simulink model "Noa_Nofusion_backup"  (R2020b)
settings: Solver=FixedStepDiscrete  StartTime=0.0  StopTime=Inf  FixedStep=0.02  RelTol=1e-3
PostLoadFcn:
  | if any(exist('dsrtsu_mdlpostloadfcn', 'file') ~= 0), dsrtsu_mdlpostloadfcn('Execute', bdroot); end
InitFcn:
  | , if any(exist('rtifpga_mdlclblib', 'file') ~= 0), rtifpga_mdlclblib('Init', bdroot); end,
  | , if any(exist('dsmpb_private', 'file') ~= 0), dsmpb_private('dsmpb_mdlclblib', 'Init', bdroot); end,
undefined symbols (not defined in the file): ACC_TimeGap_DecSetSwt, ACC_TimeGap_IncSetSwt, AccelPedalPosn, AccelPedalPosnVldty, AccelPedlPosnDiagc, AccPedalOverride, ACU_ShiftInProgress, ADAS_Posn_CurLane, AESSwtReq, ALC_SwtReq, BrkPedalSts, CC_ACC_CANCEL_OFFSwt, CC_ACC_CRUISE_OFFSwt, CC_ACC_DecSetSpd_SetSwt, CC_ACC_IncSetSpd_ResuSwt, CC_ACCSwtErr, CharSpd_ms, CSA_NODE, CURRENT_GEAR, CurrentGearValid, DiscIntNeverNeededParam, DrvDoorSts, DrvSBR, DrvTrqReqOvld, ECMACCInterface, ECMRespACC, ELKSwtReq, EngLimpHomeSts, EngSpd, EngState, EngState_PHEV, EngTrqMaxActSpd, EngTrqMinAct, EPS_DrvInpTrqVal_HighReslolution, EPS_FailSts, EPS_LKATorqOvrlDlvd, EPS_LKATorqOvrlDlvdVld, EPS_LKATrqOvlDlvdSts, EPS_SteerMod, EPS_TrqSnsrSts, EQ4_APPINFO, EQ4_LA_ELEM, EQ4_LA_HDR, EQ4_LAP_ELEM, EQ4_LAP_HDR, EQ4_LH_ELEM, EQ4_LH_HDR, EQ4_LRE_ELEM, EQ4_LRE_HDR, ESS_PedSwtReq, ESS_VehSwtReq, FFogLmpSts_F_Pbox, FLWheelDriveDirection, FLWheelSpd, FrntWiprSwtSts, FrntWshrSwtSts, FRWheelDriveDirection, FRWheelSpd, HazardLmpSwtSts, HCU_AccelPedalPosn_Diag ... (+152)
libraries: simulink x117, dsmpblib x30
(part 7 of 11)

== system Noa_Nofusion_backup/Common/Subsystem7/DS ==
  canDMSSts : Inport  OutDataTypeStr=uint8
  canHeadDetn : Inport  Port=2  OutDataTypeStr=boolean
  canDistrctnLevel : Inport  Port=3  OutDataTypeStr=uint8
  canDistrctnQlty : Inport  Port=4  OutDataTypeStr=uint8
  canDrowsnsLevel : Inport  Port=5  OutDataTypeStr=uint8
  DriverStsConditnJudge : Subsystem
  DriverSts_StateMachine : Stateflow chart  TreatAsAtomicUnit=on
  P_DMS_tDSGoodUnbeliv2LowDistrctn : Constant  Value=P_DMS_tDSGoodUnbeliv2LowDistrctn
  P_DMS_tDSGoodUnbeliv2LowDrowsns : Constant  Value=P_DMS_tDSGoodUnbeliv2LowDrowsns
  P_DMS_tDSGoodUnbeliv2MidDistractn : Constant  Value=P_DMS_tDSGoodUnbeliv2MidDistractn
  P_DMS_tDSGoodUnbeliv2MidDrowsns : Constant  Value=P_DMS_tDSGoodUnbeliv2MidDrowsns
  P_DMS_tDSLow2MidDistractn : Constant  Value=P_DMS_tDSLow2MidDistractn
  P_DMS_tDSLow2MidDrowsns : Constant  Value=P_DMS_tDSLow2MidDrowsns
  P_DMS_tDSOther2Hi1Distractn : Constant  Value=P_DMS_tDSOther2Hi1Distractn
  P_DMS_tDSOther2Hi1Drowsns : Constant  Value=P_DMS_tDSOther2Hi1Drowsns
  P_DMS_tDSOther2Hi2Distractn : Constant  Value=P_DMS_tDSOther2Hi2Distractn
  P_DMS_tDSOther2Hi2Drowsns : Constant  Value=P_DMS_tDSOther2Hi2Drowsns
  DistractnSts : Outport  OutDataTypeStr=uint8
  DrowsnsSts : Outport  Port=2  OutDataTypeStr=uint8
  DriverSts : Outport  Port=3  OutDataTypeStr=uint8
  wires:
  canDistrctnLevel/1 -> DriverStsConditnJudge/3(canDistrctnLevel)
  canDistrctnQlty/1 -> DriverStsConditnJudge/4(canDistrctnQlty)
  canHeadDetn/1 -> DriverStsConditnJudge/2(canHeadDetn)
  canDrowsnsLevel/1 -> DriverStsConditnJudge/5(canDrowsnsLevel)
  canDMSSts/1 -> DriverStsConditnJudge/1(canDMSSts)
  P_DMS_tDSGoodUnbeliv2LowDistrctn/1 -> DriverStsConditnJudge/6(PtDSGoodUnbeliv2LowDistrctn)
  P_DMS_tDSGoodUnbeliv2MidDistractn/1 -> DriverStsConditnJudge/7(PtDSGoodUnbeliv2MidDistractn)
  P_DMS_tDSLow2MidDistractn/1 -> DriverStsConditnJudge/8(PtDSLow2MidDistractn)
  P_DMS_tDSOther2Hi1Distractn/1 -> DriverStsConditnJudge/9(PtDSOther2Hi1Distractn)
  P_DMS_tDSOther2Hi2Distractn/1 -> DriverStsConditnJudge/10(PtDSOther2Hi2Distractn)
  P_DMS_tDSGoodUnbeliv2LowDrowsns/1 -> DriverStsConditnJudge/11(PtDSGoodUnbeliv2LowDrowsns)
  P_DMS_tDSGoodUnbeliv2MidDrowsns/1 -> DriverStsConditnJudge/12(PtDSGoodUnbeliv2MidDrowsns)
  P_DMS_tDSLow2MidDrowsns/1 -> DriverStsConditnJudge/13(PtDSLow2MidDrowsns)
  P_DMS_tDSOther2Hi1Drowsns/1 -> DriverStsConditnJudge/14(PtDSOther2Hi1Drowsns)
  P_DMS_tDSOther2Hi2Drowsns/1 -> DriverStsConditnJudge/15(PtDSOther2Hi2Drowsns)
  DriverStsConditnJudge/1(DSOther2Good) -> DriverSts_StateMachine/1(DSOther2Good)
  DriverStsConditnJudge/2(DSOther2Unbeliv) -> DriverSts_StateMachine/2(DSOther2Unbeliv)
  DriverStsConditnJudge/3(DSGoodUnbeliv2LowDistractn) -> DriverSts_StateMachine/3(DSGoodUnbeliv2LowDistractn)
  DriverStsConditnJudge/4(DSMidHi1Hi22LowDistractn) -> DriverSts_StateMachine/4(DSMidHi1Hi22LowDistractn)
  DriverStsConditnJudge/5(DSGoodUnbeliv2MidDistractn) -> DriverSts_StateMachine/5(DSGoodUnbeliv2MidDistractn)
  DriverStsConditnJudge/6(DSLow2MidDistractn) -> DriverSts_StateMachine/6(DSLow2MidDistractn)
  DriverStsConditnJudge/7(DSHi1Hi22MidDistractn) -> DriverSts_StateMachine/7(DSHi1Hi22MidDistractn)
  DriverStsConditnJudge/8(DSOther2Hi1Distractn) -> DriverSts_StateMachine/8(DSOther2Hi1Distractn)
  DriverStsConditnJudge/9(DSOther2Hi2Distractn) -> DriverSts_StateMachine/9(DSOther2Hi2Distractn)
  DriverStsConditnJudge/10(DSGoodUnbeliv2LowDrowsns) -> DriverSts_StateMachine/10(DSGoodUnbeliv2LowDrowsns)
  DriverStsConditnJudge/11(DSMidHi1Hi22LowDrowsns) -> DriverSts_StateMachine/11(DSMidHi1Hi22LowDrowsns)
  DriverStsConditnJudge/12(DSGoodUnbeliv2MidDrowsns) -> DriverSts_StateMachine/12(DSGoodUnbeliv2MidDrowsns)
  DriverStsConditnJudge/13(DSLow2MidDrowsns) -> DriverSts_StateMachine/13(DSLow2MidDrowsns)
  DriverStsConditnJudge/14(DSHi1Hi22MidDrowsns) -> DriverSts_StateMachine/14(DSHi1Hi22MidDrowsns)
  DriverStsConditnJudge/15(DSOther2Hi1Drowsns) -> DriverSts_StateMachine/15(DSOther2Hi1Drowsns)
  DriverStsConditnJudge/16(DSOther2Hi2Drowsns) -> DriverSts_StateMachine/16(DSOther2Hi2Drowsns)
  DriverStsConditnJudge/17(DSMidHi1Hi22NoDistractn) -> DriverSts_StateMachine/17(DSMidHi1Hi22NoDistractn)
  DriverStsConditnJudge/18(DSMidHi1Hi22NoDrowsns) -> DriverSts_StateMachine/18(DSMidHi1Hi22NoDrowsns)
  DriverStsConditnJudge/19(DSUnbeliv2DDAEnable) -> DriverSts_StateMachine/19(DSUnbeliv2DDAEnable)
  DriverSts_StateMachine/1(DistractnSts) -> DistractnSts/1
  DriverSts_StateMachine/2(DrowsnsSts) -> DrowsnsSts/1
  DriverSts_StateMachine/3(DriverSts) -> DriverSts/1

== system Noa_Nofusion_backup/LPV/Subsystem5/For Each Subsystem1 ==
  In1 : Inport  Partition=on  PartitionDimension=1  PartitionWidth=1  PartitionOffset=0
  Bus Assignment4 : BusAssignment  AssignedSignals=LH_CRC,LH_Is_Triggered_SDM_Type,LH_Is_Triggered_SDM_Model,LH_Track_ID,LH_Age,LH_Confidence,Reserved_3,LH_Prediction_Reason,LH_Availability_State,LH_Color,LH_Color_Confidence,LH_Lanemark_Type,LH_DLM_Type,LH_DECEL_Type,Reserved_4,LH_Lanemark_Type_Conf,LH_Side,LH_Crossing,LH_Marker_Width,LH_Marker_Width_STD,Reserved_5,LH_Dash_Average_Length,LH_Dash_Average_Gap,LH_Is_Multi_Clothoid,Reserved_6,LH_Line_First_C0,LH_Line_First_C1,LH_Line_First_C2,LH_Line_First_C3,LH_First_VR_Start,LH_First_VR_End,Reserved_7,LH_First_Measured_VR_End,LH_Second_Measured_VR_End,Reserved_8,LH_Line_Second_C0,LH_Line_Second_C1,LH_Line_Second_C2,LH_Line_Second_C3,LH_Second_VR_Start,LH_Second_VR_End,LH_Buffer_C3
  Bus Selector : BusSelector  OutputSignals=LH_CRC,LH_Is_Triggered_SDM_Type,LH_Is_Triggered_SDM_Model,LH_Track_ID,LH_Age,LH_Confidence,Reserved_3,LH_Prediction_Reason,LH_Availability_State,LH_Color,LH_Color_Confidence,LH_Lanemark_Type,LH_DLM_Type,LH_DECEL_Type,Reserved_4,LH_Lanemark_Type_Conf,LH_Side,LH_Crossing,LH_Marker_Width,LH_Marker_Width_STD,Reserved_5,LH_Dash_Average_Length,LH_Dash_Average_Gap,LH_Is_Multi_Clothoid,Reserved_6,LH_Line_First_C0,LH_Line_First_C1,LH_Line_First_C2,LH_Line_First_C3,LH_First_VR_Start,LH_First_VR_End,Reserved_7,LH_First_Measured_VR_End,LH_Second_Measured_VR_End,Reserved_8,LH_Line_Second_C0,LH_Line_Second_C1,LH_Line_Second_C2,LH_Line_Second_C3,LH_Second_VR_Start,LH_Second_VR_End,LH_Buffer_C3
  Constant4 : Constant  Value=0  OutDataTypeStr=Bus: EQ4_LH_ELEM_BUS
  For Each : ForEach  DisableCoverage=on
  Out1 : Outport  ConcatenationDimension=1
  wires:
  Bus Selector/42 -> Bus Assignment4/43  "<LH_Buffer_C3>"
  Bus Selector/41 -> Bus Assignment4/42  "<LH_Second_VR_End>"
  Bus Selector/40 -> Bus Assignment4/41  "<LH_Second_VR_Start>"
  Bus Selector/39 -> Bus Assignment4/40  "<LH_Line_Second_C3>"
  Bus Selector/38 -> Bus Assignment4/39  "<LH_Line_Second_C2>"
  Bus Selector/37 -> Bus Assignment4/38  "<LH_Line_Second_C1>"
  Bus Selector/36 -> Bus Assignment4/37  "<LH_Line_Second_C0>"
  Bus Selector/35 -> Bus Assignment4/36  "<Reserved_8>"
  Bus Selector/34 -> Bus Assignment4/35  "<LH_Second_Measured_VR_End>"
  Bus Selector/33 -> Bus Assignment4/34  "<LH_First_Measured_VR_End>"
  Bus Selector/32 -> Bus Assignment4/33  "<Reserved_7>"
  Bus Selector/31 -> Bus Assignment4/32  "<LH_First_VR_End>"
  Bus Selector/30 -> Bus Assignment4/31  "<LH_First_VR_Start>"
  Bus Selector/29 -> Bus Assignment4/30  "<LH_Line_First_C3>"
  Bus Selector/28 -> Bus Assignment4/29  "<LH_Line_First_C2>"
  Bus Selector/27 -> Bus Assignment4/28  "<LH_Line_First_C1>"
  Bus Selector/26 -> Bus Assignment4/27  "<LH_Line_First_C0>"
  Bus Selector/25 -> Bus Assignment4/26  "<Reserved_6>"
  Bus Selector/24 -> Bus Assignment4/25  "<LH_Is_Multi_Clothoid>"
  Bus Selector/23 -> Bus Assignment4/24  "<LH_Dash_Average_Gap>"
  Bus Selector/22 -> Bus Assignment4/23  "<LH_Dash_Average_Length>"
  Bus Selector/21 -> Bus Assignment4/22  "<Reserved_5>"
  Bus Selector/20 -> Bus Assignment4/21  "<LH_Marker_Width_STD>"
  Bus Selector/19 -> Bus Assignment4/20  "<LH_Marker_Width>"
  Bus Selector/18 -> Bus Assignment4/19  "<LH_Crossing>"
  Bus Selector/17 -> Bus Assignment4/18  "<LH_Side>"
  Bus Selector/16 -> Bus Assignment4/17  "<LH_Lanemark_Type_Conf>"
  Bus Selector/15 -> Bus Assignment4/16  "<Reserved_4>"
  Bus Selector/14 -> Bus Assignment4/15  "<LH_DECEL_Type>"
  Bus Selector/13 -> Bus Assignment4/14  "<LH_DLM_Type>"
  Bus Selector/12 -> Bus Assignment4/13  "<LH_Lanemark_Type>"
  Bus Selector/11 -> Bus Assignment4/12  "<LH_Color_Confidence>"
  Bus Selector/10 -> Bus Assignment4/11  "<LH_Color>"
  Bus Selector/9 -> Bus Assignment4/10  "<LH_Availability_State>"
  Bus Selector/8 -> Bus Assignment4/9  "<LH_Prediction_Reason>"
  Bus Selector/7 -> Bus Assignment4/8  "<Reserved_3>"
  Bus Selector/6 -> Bus Assignment4/7  "<LH_Confidence>"
  Bus Selector/5 -> Bus Assignment4/6  "<LH_Age>"
  Bus Selector/4 -> Bus Assignment4/5  "<LH_Track_ID>"
  Bus Selector/3 -> Bus Assignment4/4  "<LH_Is_Triggered_SDM_Model>"
  Bus Selector/2 -> Bus Assignment4/3  "<LH_Is_Triggered_SDM_Type>"
  Bus Selector/1 -> Bus Assignment4/2  "<LH_CRC>"
  Bus Assignment4/1 -> Out1/1
  In1/1 -> Bus Selector/1
  Constant4/1 -> Bus Assignment4/1

== system Noa_Nofusion_backup/LPV/Subsystem5/For Each Subsystem2 ==
  In1 : Inport  Partition=on  PartitionDimension=1  PartitionWidth=1  PartitionOffset=0
  Bus Assignment4 : BusAssignment  AssignedSignals=LRE_ID,LRE_Age,LRE_Confidence,LRE_Type,Reserved_2,LRE_Prediction_Reason,LRE_Availability_State,LRE_Height,LRE_Height_STD,Reserved_3,LRE_View_Range_Start,LRE_View_Range_End,Reserved_4,LRE_Measured_VR_End,LRE_Side,LRE_Is_Triggered_SDM_Model,Reserved_5,LRE_Line_C3,LRE_Line_C2,LRE_Line_C1,LRE_Line_C0,LRE_Detection_Source,Reserved_6
  Bus Selector : BusSelector  OutputSignals=LRE_ID,LRE_Age,LRE_Confidence,LRE_Type,Reserved_2,LRE_Prediction_Reason,LRE_Availability_State,LRE_Height,LRE_Height_STD,Reserved_3,LRE_View_Range_Start,LRE_View_Range_End,Reserved_4,LRE_Measured_VR_End,LRE_Side,LRE_Is_Triggered_SDM_Model,Reserved_5,LRE_Line_C3,LRE_Line_C2,LRE_Line_C1,LRE_Line_C0,LRE_Detection_Source,Reserved_6
  Constant4 : Constant  Value=0  OutDataTypeStr=Bus: EQ4_LRE_ELEM_BUS
  For Each : ForEach  DisableCoverage=on
  Out1 : Outport  ConcatenationDimension=1
  wires:
  Bus Selector/23 -> Bus Assignment4/24  "<Reserved_6>"
  Bus Selector/22 -> Bus Assignment4/23  "<LRE_Detection_Source>"
  Bus Selector/21 -> Bus Assignment4/22  "<LRE_Line_C0>"
  Bus Selector/20 -> Bus Assignment4/21  "<LRE_Line_C1>"
  Bus Selector/19 -> Bus Assignment4/20  "<LRE_Line_C2>"
  Bus Selector/18 -> Bus Assignment4/19  "<LRE_Line_C3>"
  Bus Selector/17 -> Bus Assignment4/18  "<Reserved_5>"
  Bus Selector/16 -> Bus Assignment4/17  "<LRE_Is_Triggered_SDM_Model>"
  Bus Selector/15 -> Bus Assignment4/16  "<LRE_Side>"
  Bus Selector/14 -> Bus Assignment4/15  "<LRE_Measured_VR_End>"
  Bus Selector/13 -> Bus Assignment4/14  "<Reserved_4>"
  Bus Selector/12 -> Bus Assignment4/13  "<LRE_View_Range_End>"
  Bus Selector/11 -> Bus Assignment4/12  "<LRE_View_Range_Start>"
  Bus Selector/10 -> Bus Assignment4/11  "<Reserved_3>"
  Bus Selector/9 -> Bus Assignment4/10  "<LRE_Height_STD>"
  Bus Selector/8 -> Bus Assignment4/9  "<LRE_Height>"
  Bus Selector/7 -> Bus Assignment4/8  "<LRE_Availability_State>"
  Bus Selector/6 -> Bus Assignment4/7  "<LRE_Prediction_Reason>"
  Bus Selector/5 -> Bus Assignment4/6  "<Reserved_2>"
  Bus Selector/4 -> Bus Assignment4/5  "<LRE_Type>"
  Bus Selector/3 -> Bus Assignment4/4  "<LRE_Confidence>"
  Bus Selector/2 -> Bus Assignment4/3  "<LRE_Age>"
  Bus Selector/1 -> Bus Assignment4/2  "<LRE_ID>"
  Constant4/1 -> Bus Assignment4/1
  In1/1 -> Bus Selector/1
  Bus Assignment4/1 -> Out1/1

== system Noa_Nofusion_backup/LPV/Subsystem5/For Each Subsystem3 ==
  In1 : Inport  Partition=on  PartitionDimension=1  PartitionWidth=1  PartitionOffset=0
  Bus Assignment4 : BusAssignment  AssignedSignals=LA_Lane_Track_ID,LA_Age,LA_Confidence,LA_Color,LA_Color_Conf,LA_Prediction_Reason,LA_Availability_State,LA_View_Range_Start,Reserved_2,LA_View_Range_End,LA_Measured_VR_End,Reserved_3,LA_Lanemark_Type,LA_DLM_Type,LA_Lanemark_Type_Conf,LA_Line_Side,LA_Marker_Width,Reserved_4,LA_Marker_Width_STD,Reserved_5,LA_Line_C3,LA_Line_C2,LA_Line_C1,LA_Line_C0,LH_Buffer_C1,Reserved_6
  Bus Selector : BusSelector  OutputSignals=LA_Lane_Track_ID,LA_Age,LA_Confidence,LA_Color,LA_Color_Conf,LA_Prediction_Reason,LA_Availability_State,LA_View_Range_Start,Reserved_2,LA_View_Range_End,LA_Measured_VR_End,Reserved_3,LA_Lanemark_Type,LA_DLM_Type,LA_Lanemark_Type_Conf,LA_Line_Side,LA_Marker_Width,Reserved_4,LA_Marker_Width_STD,Reserved_5,LA_Line_C3,LA_Line_C2,LA_Line_C1,LA_Line_C0,LH_Buffer_C1,Reserved_6
  Constant4 : Constant  Value=0  OutDataTypeStr=Bus: EQ4_LA_ELEM_BUS
  For Each : ForEach  DisableCoverage=on
  Out1 : Outport  ConcatenationDimension=1
  wires:
  Bus Selector/26 -> Bus Assignment4/27  "<Reserved_6>"
  Bus Selector/25 -> Bus Assignment4/26  "<LH_Buffer_C1>"
  Bus Selector/24 -> Bus Assignment4/25  "<LA_Line_C0>"
  Bus Selector/23 -> Bus Assignment4/24  "<LA_Line_C1>"
  Bus Selector/22 -> Bus Assignment4/23  "<LA_Line_C2>"
  Bus Selector/21 -> Bus Assignment4/22  "<LA_Line_C3>"
  Bus Selector/20 -> Bus Assignment4/21  "<Reserved_5>"
  Bus Selector/19 -> Bus Assignment4/20  "<LA_Marker_Width_STD>"
  Bus Selector/18 -> Bus Assignment4/19  "<Reserved_4>"
  Bus Selector/17 -> Bus Assignment4/18  "<LA_Marker_Width>"
  Bus Selector/16 -> Bus Assignment4/17  "<LA_Line_Side>"
  Bus Selector/15 -> Bus Assignment4/16  "<LA_Lanemark_Type_Conf>"
  Bus Selector/14 -> Bus Assignment4/15  "<LA_DLM_Type>"
  Bus Selector/13 -> Bus Assignment4/14  "<LA_Lanemark_Type>"
  Bus Selector/12 -> Bus Assignment4/13  "<Reserved_3>"
  Bus Selector/11 -> Bus Assignment4/12  "<LA_Measured_VR_End>"
  Bus Selector/10 -> Bus Assignment4/11  "<LA_View_Range_End>"
  Bus Selector/9 -> Bus Assignment4/10  "<Reserved_2>"
  Bus Selector/8 -> Bus Assignment4/9  "<LA_View_Range_Start>"
  Bus Selector/7 -> Bus Assignment4/8  "<LA_Availability_State>"
  Bus Selector/6 -> Bus Assignment4/7  "<LA_Prediction_Reason>"
  Bus Selector/5 -> Bus Assignment4/6  "<LA_Color_Conf>"
  Bus Selector/4 -> Bus Assignment4/5  "<LA_Color>"
  Bus Selector/3 -> Bus Assignment4/4  "<LA_Confidence>"
  Bus Selector/2 -> Bus Assignment4/3  "<LA_Age>"
  Bus Selector/1 -> Bus Assignment4/2  "<LA_Lane_Track_ID>"
  Constant4/1 -> Bus Assignment4/1
  In1/1 -> Bus Selector/1
  Bus Assignment4/1 -> Out1/1

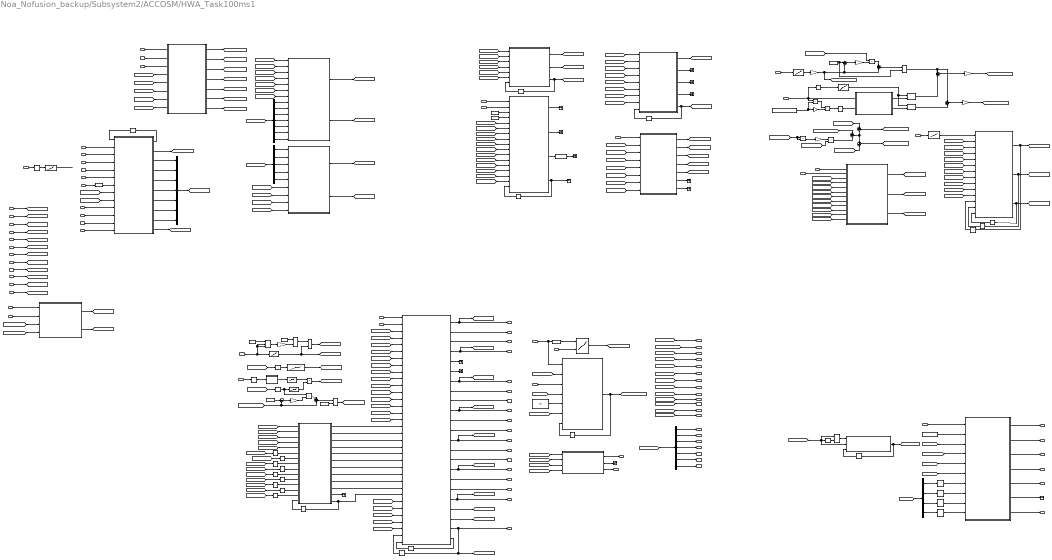
== system Noa_Nofusion_backup/Subsystem2/ACCOSM/HWA_Task100ms1 ==
  note: part03/TOS/Subsystem1/ACCOSM/HWA_Task100ms1
  note: OTL
  note: ATS
  note: PLA
  note: ASI_CalcPreOSF
  note: EIA
  note: 存在时间
  ObjRange_m : Inport
  ObjDx_m : Inport  Port=2
  ObjDy_m : Inport  Port=3
  ObjValid : Inport  Port=4
  ObjClassification : Inport  Port=5
  ObjVxG_ms : Inport  Port=6
  ObjVyG_ms : Inport  Port=7
  ObjArG_ms2 : Inport  Port=8
  ObjWidth_m : Inport  Port=9
  ObjCnt : Inport  Port=10
  ObjMoveSts : Inport  Port=11
  ObjBrakeLightIndic : Inport  Port=12
  A2 : Inport  Port=13
  A1 : Inport  Port=14
  Conf : Inport  Port=15
  TimeGap : Inport  Port=16
  ACCMode : Inport  Port=17
  VxvRef_ms : Inport  Port=18
  kapCurvTraj : Inport  Port=19
  AlpSideSlipAngle : Inport  Port=20
  AlpWheelAngle : Inport  Port=21
  alpSumSlideCurveness : Inport  Port=22
  LongitudeAcc : Inport  Port=23
  TarLineValid : Inport  Port=24
  TarLine_A2 : Inport  Port=25
  TarLine_A1 : Inport  Port=26
  TarLine_A0 : Inport  Port=27
  1-D Lookup Table1 : Lookup_n-D  NumberOfTableDimensions=1  BreakpointsForDimension1=[0,8,23,55,60]  Table=[80,80,120,200,200]  RndMeth=Simplest  InputSameDT=on
  1-D Lookup Table2 : Lookup_n-D  NumberOfTableDimensions=1  BreakpointsForDimension1=[0,0.035,0.057,0.1]  Table=[1,1,0,0]  RndMeth=Simplest  InputSameDT=on
  ACCMode1 : InportShadow  Port=17
  ACC_DisplayBar : MATLAB Function  TreatAsAtomicUnit=on
  Abs : Abs
  Abs1 : Abs
  Abs2 : Abs
  AlpSideSlipAngle_1 : InportShadow  Port=20
  Bus Creator : BusCreator  Inputs=7
  Bus Selector : BusSelector  OutputSignals=dxC0,aPC0,bPC0,cPC0,aPC1,bPC1,cPC1
  Bus Selector1 : BusSelector  OutputSignals=dxC0,aPC0,bPC0,aPC1,bPC1
  Bus Selector2 : BusSelector  OutputSignals=dxC0,aPC0,bPC0,cPC0,aPC1,bPC1,cPC1
  Bus Selector3 : BusSelector  OutputSignals=dDeltaX,dDeltaY,CosOfPsi,SinOfPsi
  Compare To Constant : simulink/Logic and Bit Operations/Compare To Constant  relop=>=  const=1  OutDataTypeStr=boolean
  Compare To Constant1 : simulink/Logic and Bit Operations/Compare To Constant  relop=>=  const=0.7  OutDataTypeStr=boolean
  Constant : Constant  Value=15  OutDataTypeStr=single
  Constant1 : Constant  Value=0.6  OutDataTypeStr=single
  Constant3 : Constant  Value=[0.6,0.75,0.9;0.58,0.68,0.77;0.41,0.55,0.63;0.38,0.44,0.49]  OutDataTypeStr=single
  Constant6 : Constant  Value=0.1  OutDataTypeStr=single
  Data Type Conversion7 : DataTypeConversion  OutDataTypeStr=single
  DeltaDx : Lookup_n-D  NumberOfTableDimensions=1  BreakpointsForDimension1=[0,30,60,100,120,130]  Table=[2,4,6,8,9,9]  RndMeth=Simplest  InputSameDT=on
  DeltaDy : Lookup_n-D  NumberOfTableDimensions=1  BreakpointsForDimension1=[0,30,60,100,120,130]  Table=[0.5,0.5,1,1.2,1.5,1.5]  RndMeth=Simplest  InputSameDT=on
  DesireDistance : Lookup_n-D  BreakpointsForDimension1=[1,2,3,4]  BreakpointsForDimension2=[0,2.6,17,25,35,60]  BreakpointsForDimension1DataTypeStr=single  BreakpointsForDimension2DataTypeStr=single  Table=reshape([4,4.3,4.6,4.9,7.8,8.5,9,9.5,18,23,28,34,27,37,47,54,35,49,63,71,60,70,80,85],4,6)  TableDataTypeStr=single  RndMeth=Simplest
      settings: InputPortMap=u0,u1
  Dyc : MATLAB Function  TreatAsAtomicUnit=on
  DycCutIn : MATLAB Function  TreatAsAtomicUnit=on
  DycHistCalc : MATLAB Function  TreatAsAtomicUnit=on
  Fac : Lookup_n-D  NumberOfTableDimensions=1  BreakpointsForDimension1=[0,0.4,0.6,0.8]  Table=[1,1,1.5,1.5]  RndMeth=Simplest  InputSameDT=on
  Gain{,1,3..4} (4 alike) : Gain  Gain=0.5
  Gain2 : Gain  Gain=0.95
  Gain5 : Gain  Gain=0.02
  Gain6 : Gain  Gain=0.95
  Gain8 : Gain  Gain=0.02
  LostTargetCalc : MATLAB Function  TreatAsAtomicUnit=on
  Lpb : MATLAB Function  TreatAsAtomicUnit=on
  Memory{1..2,4,6,13..14} (6 alike) : Memory  InitialCondition=single(zeros(15,1))  InheritSampleTime=on
  Memory10 : Memory  InitialCondition=uint8(0)  InheritSampleTime=on
  Memory12 : Memory  InheritSampleTime=on
  Memory{8,15..16,18..22,25,27..28} (11 alike) : Memory  InitialCondition=single(0)  InheritSampleTime=on
  Memory17 : Memory  InitialCondition=uint8(0)  InheritSampleTime=on
  Memory24 : Memory  InitialCondition=false  InheritSampleTime=on
  Memory26 : Memory  InitialCondition=false  InheritSampleTime=on
  Memory3 : Memory  InheritSampleTime=on
  Memory30 : Memory  InitialCondition=uint8(0)  InheritSampleTime=on
  MinMax : MinMax  Function=max  Inputs=2
  MinMax1 : MinMax  Function=max  Inputs=2
  MinMax2 : MinMax  Inputs=2
  MinMax4 : MinMax  Inputs=2
  MinMax5 : MinMax  Function=max  Inputs=2
  MinMax6 : MinMax  Inputs=2
  OTL1 : Subsystem
  Plaus : MATLAB Function  TreatAsAtomicUnit=on
  Product{,1..6} (7 alike) : Product
  Product7 : Product  Inputs=/**
  Relational Operator1 : RelationalOperator  Operator===  OutDataTypeStr=boolean  RndMeth=Nearest
  Signal Copy{,1..3} (4 alike) : SignalConversion  OverrideOpt=off
  Spw : MATLAB Function  TreatAsAtomicUnit=on
  Std : MATLAB Function  TreatAsAtomicUnit=on
  Sum1 : Sum  Inputs=|+-
  Sum10 : Sum  Inputs=-+
  Sum11 : Sum  Inputs=|+-
  Sum{2..4,13} (4 alike) : Sum
  Sum8 : Sum  Inputs=+-
  Sum9 : Sum  Inputs=+-
  Tapped Delay : simulink/Discrete/Tapped Delay  vinit=0.0  samptime=-1  NumDelays=4  DelayOrder=Newest  includeCurrent=on
  TargetBrake : MATLAB Function  TreatAsAtomicUnit=on
  TargetSelect : MATLAB Function  TreatAsAtomicUnit=on
  Terminator{,1,3,9..15,17..20} (14 alike) : Terminator
  TimeCalc : MATLAB Function  TreatAsAtomicUnit=on
  Trajectory : Subsystem  TreatAsAtomicUnit=on
  VxVy : Subsystem
  VxvRef_ms_{1..10} (10 alike) : InportShadow  Port=18
  VycCalc : MATLAB Function  TreatAsAtomicUnit=on
  alpSumSlideCurveness1 : InportShadow  Port=22
  dxMaxFollowPO : Lookup_n-D  NumberOfTableDimensions=1  BreakpointsForDimension1=[8.33,22.22,37.5]  Table=[90,120,120]  InternalRulePriority=Speed  RndMeth=Simplest  InputSameDT=on
  dyLaneWidthMin : Lookup_n-D  NumberOfTableDimensions=1  BreakpointsForDimension1=[0,2.78,8.33,10]  Table=[3,3,2.8,2.8]  InternalRulePriority=Speed  RndMeth=Simplest  InputSameDT=on
  dyLaneWidthMinHalfStatObj1 : Constant  Value=P_Global_DxvFrontBumper_m  OutDataTypeStr=single
  dyLaneWidthMinHalfStatObj10 : Constant  Value=2.2  OutDataTypeStr=single
  dyLaneWidthMinHalfStatObj2 : Constant  Value=2.2  OutDataTypeStr=single
  dyLaneWidthMinHalfStatObj5 : Constant  Value=0  OutDataTypeStr=single
  dyLaneWidthMinHalfStatObj7 : Constant  Value=0  OutDataTypeStr=single
  dyLaneWidthMinHalfStatObj9 : Constant  Value=2.2  OutDataTypeStr=single
  dyLaneWidthSteerAdapt : MATLAB Function  TreatAsAtomicUnit=on
  kapCurvTraj_{1..4} (4 alike) : InportShadow  Port=19
  t_dyLaneWidthSteerAdapt : Lookup_n-D  NumberOfTableDimensions=1  BreakpointsForDimension1=[0,0.02,0.05,0.1]  Table=[0,0,0.7,0.7]  InternalRulePriority=Speed  RndMeth=Simplest  InputSameDT=on
  wCutInVy : MATLAB Function  TreatAsAtomicUnit=on
  wCutOutVy : MATLAB Function  TreatAsAtomicUnit=on
  P0ID : Outport
  P2ID : Outport  Port=2
  P3ID : Outport  Port=3
  TargetBrake_b : Outport  Port=4
  P0Range : Outport  Port=5
  P0Vr : Outport  Port=6
  P2Vr : Outport  Port=7
  P3Vr : Outport  Port=8
  P0ArG : Outport  Port=9
  P2ArG : Outport  Port=10
  P3ArG : Outport  Port=11
  P0Dx : Outport  Port=12
  P2Dx : Outport  Port=13
  P3Dx : Outport  Port=14
  P0Dy : Outport  Port=15
  P2Dy : Outport  Port=16
  P3Dy : Outport  Port=17
  CutIn_b : Outport  Port=18
  TargetExist : Outport  Port=19
  DesireDis : Outport  Port=20
  Signal_ACC_TgtObjBarDisp : Outport  Port=21
  ObjDyc_m : Outport  Port=22
  ObjVy_ms : Outport  Port=23
  ObjVyc_ms : Outport  Port=24
  ObjSpw : Outport  Port=25
  ObjSpwLeft : Outport  Port=26
  ObjSpwRight : Outport  Port=27
  ObjPlaus : Outport  Port=28
  ObjPlausLeft : Outport  Port=29
  ObjPlausRight : Outport  Port=30
  ObjDycHist : Outport  Port=31
  ObjqDycHist : Outport  Port=32
  dxC0 : Outport  Port=33
  aPC0 : Outport  Port=34
  bPC0 : Outport  Port=35
  cPC0 : Outport  Port=36
  aPC1 : Outport  Port=37
  bPC1 : Outport  Port=38
  cPC1 : Outport  Port=39
  OTLValid : Outport  Port=40
  aOTL : Outport  Port=41
  bOTL : Outport  Port=42
  cOTL : Outport  Port=43
  dOTL : Outport  Port=44
  dxMaxOTL : Outport  Port=45
  TargetVyG : Outport  Port=46
  wires:
  Signal Copy1/1 -> OTL1/10(EgoSinOfPsi)  "OTL_IN_SinOfPsi"
  Signal Copy2/1 -> OTL1/9(EgoCosOfPsi)  "OTL_IN_CosOfPsi"
  Signal Copy/1 -> OTL1/8(EgoDDeltaY)  "OTL_IN_dDeltaY"
  Signal Copy3/1 -> OTL1/7(EgoDDeltaX)  "OTL_IN_dDeltaX"
  Bus Selector3/2 -> Signal Copy/1  "<dDeltaY>"
  VxvRef_ms_10/1 -> OTL1/1(vRef)  "OTL_IN_VxvRef_ms_10"
  [TargetCutIn_b] -> OTL1/4(CutIn)  "OTL_IN_TargetCutIn_b"
  Gain6/1 -> [dyLaneWidthRight]
  Gain2/1 -> [dyLaneWidthLeft]
  TarLine_A0/1 -> Dyc/13(TarLineA0)
  OTL1/6(dxMin) -> Terminator/1  "OTL_OUT_dxMin"
  OTL1/7(dxMax) -> dxMaxOTL/1  "OTL_OUT_dxMax"
  OTL1/5(d) -> dOTL/1  "OTL_OUT_C0"
  OTL1/4(c) -> cOTL/1  "OTL_OUT_C1"
  OTL1/3(b) -> bOTL/1  "OTL_OUT_C2"
  OTL1/2(a) -> aOTL/1  "OTL_OUT_C3"
  OTL1/1(LineValid) -> OTLValid/1  "OTL_OUT_OTLValid"
  [EgoMove] -> Bus Selector3/1
  [TargetDx] -> OTL1/5(P0Dx)  "OTL_IN_TargetDx"
  Bus Selector3/1 -> Signal Copy3/1  "<dDeltaX>"
  Bus Selector3/3 -> Signal Copy2/1  "<CosOfPsi>"
  [tSameHandleT1] -> OTL1/3(tSameHandle)
  [TargetDy] -> OTL1/6(P0Dy)  "OTL_IN_TargetDy"
  Bus Selector3/4 -> Signal Copy1/1  "<SinOfPsi>"
  Constant6/1 -> OTL1/2(tCycle)
  Trajectory/7(EgoMove) -> [EgoMove]
  Memory12/1 -> Relational Operator1/2
  Memory3/1 -> TimeCalc/3(tSameHandleTK1)
  TimeCalc/1(tSameHandleT) -> [tSameHandleT1], Memory3/1
  Relational Operator1/1 -> TimeCalc/1(SameTarget)
  [TargetID] -> TimeCalc/2(TargetID), Memory12/1, Relational Operator1/1  "OTL_IN_TargetID"
  TargetBrake/2(TargetVxG) -> Terminator3/1
  [ObjVxG_ms] -> TargetBrake/2(VxG)
  TargetBrake/3(TargetVyG) -> TargetVyG/1
  [ObjVyG_ms] -> TargetBrake/3(VyG)
  Compare To Constant1/1 -> Terminator1/1
  TarLine_A2/1 -> Dyc/11(TarLineA2)
  TarLineValid/1 -> Dyc/10(TarLineValid)
  TarLine_A1/1 -> Dyc/12(TarLineA1)
  [TrajHistBufferDyv] -> DycHistCalc/6(TrajHistBufferDyv)
  [TrajHistBufferDxv] -> DycHistCalc/5(TrajHistBufferDxv)
  [TrajHistBufferBValid] -> DycHistCalc/4(TrajHistBufferBValid)
  [TrajCurrentIndex] -> DycHistCalc/3(TrajCurrentIndex)
  [ObjTrajNumber] -> DycHistCalc/2(ObjTrajNumber)
  [TrajHistBufferBTrajEnd] -> DycHistCalc/1(TrajHistBufferBTrajEnd)
  Trajectory/6(Out13) -> [TrajHistBufferDyv]
  Trajectory/5(Out12) -> [TrajHistBufferDxv]
  Trajectory/4(Out11) -> [TrajHistBufferBValid]
  Trajectory/3(Out10) -> [TrajCurrentIndex]
  Trajectory/2(Out9) -> [ObjTrajNumber]
  Trajectory/1(Out8) -> [TrajHistBufferBTrajEnd]
  [ObjCnt] -> TargetSelect/11(Cnt)
  MinMax6/1 -> [TarLimS0Dx]
  Constant1/1 -> Product7/1
  [TarLimS0Dx] -> TargetSelect/32(TarLimS0Dx)
  MinMax5/1 -> MinMax6/1
  Product7/1 -> Gain1/1
  Gain1/1 -> MinMax5/2
  1-D Lookup Table1/1 -> [TarLimDx], MinMax6/2
  VxvRef_ms_4/1 -> 1-D Lookup Table1/1, Product7/3, Product7/2  "OTL_IN_VxvRef_ms_10"
  Constant/1 -> MinMax5/1
  VxvRef_ms_2/1 -> DesireDistance/2  "OTL_IN_VxvRef_ms_10"
  TargetBrake/1(TargetBrake_b) -> TargetBrake_b/1
  ObjBrakeLightIndic/1 -> [ObjBrakeLightIndic]
  [ObjBrakeLightIndic] -> TargetBrake/4(BrakeLightIndic)
  [TargetID] -> TargetBrake/1(ID)
  A1/1 -> Dyc/6(A1)
  A2/1 -> Dyc/5(A2)
  [ObjDycHist] -> ObjDycHist/1
  [ObjqDycHist] -> ObjqDycHist/1
  Spw/7(ObjDyKapErr) -> Terminator13/1
  Spw/6(ObjDycASI) -> Terminator12/1
  Bus Selector2/7 -> cPC1/1  "<cPC1>"
  Bus Selector2/6 -> bPC1/1  "<bPC1>"
  Bus Selector2/5 -> aPC1/1  "<aPC1>"
  Bus Selector2/4 -> cPC0/1  "<cPC0>"
  Bus Selector2/3 -> bPC0/1  "<bPC0>"
  Bus Selector2/2 -> aPC0/1  "<aPC0>"
  Bus Selector2/1 -> dxC0/1  "<dxC0>"
  [EgoLine] -> Bus Selector2/1
  TargetSelect/6(P3Range) -> Terminator11/1
  TargetSelect/5(P2Range) -> Terminator10/1
  [ObjPlausRight] -> ObjPlausRight/1
  [ObjPlausLeft] -> ObjPlausLeft/1
  [ObjPlaus] -> ObjPlaus/1
  [ObjSpwRight] -> ObjSpwRight/1
  [ObjSpwLeft] -> ObjSpwLeft/1
  [ObjSpw] -> ObjSpw/1
  [ObjVyc] -> ObjVyc_ms/1
  LostTargetCalc/11(Covered_b) -> Terminator9/1
  [dyLaneWidth] -> TargetSelect/28(dyLaneWidth)
  LostTargetCalc/10(TargetLost_b) -> TargetSelect/26(TargetLost_b)
  LostTargetCalc/9(ReVyc) -> TargetSelect/25(ReVyc)
  LostTargetCalc/8(ReDyc) -> TargetSelect/24(ReDyc)
  LostTargetCalc/7(ReCutIn_b) -> TargetSelect/23(ReCutIn_b)
  LostTargetCalc/6(ReVx) -> TargetSelect/22(ReVx)
  LostTargetCalc/5(ReDy) -> TargetSelect/21(ReDy)
  LostTargetCalc/4(ReDx) -> TargetSelect/20(ReDx)
  LostTargetCalc/3(ReArG) -> TargetSelect/19(ReArG)
  LostTargetCalc/2(ReRange) -> TargetSelect/18(ReRange)
  LostTargetCalc/1(ReID) -> TargetSelect/17(ReID)
  dyLaneWidthMinHalfStatObj10/1 -> MinMax4/2
  [DeltaDy] -> LostTargetCalc/5(DeltaDy)
  [DeltaDx] -> LostTargetCalc/4(DeltaDx)
  [DesireDistanceChar] -> ACC_DisplayBar/2(DesireDistance)
  Tapped Delay/1 -> Std/1(u)
  Fac/1 -> Product5/1
  Std/1(y) -> Fac/1
  [TargetDx] -> Memory15/1
  LongitudeAcc/1 -> Tapped Delay/1
  DeltaDx/1 -> Product5/2
  Product5/1 -> [DeltaDx]
  [TargetDy] -> Memory16/1
  Memory16/1 -> DeltaDy/1
  DeltaDy/1 -> [DeltaDy]
  Memory30/1 -> TargetSelect/34(TargetReplacedCntK1)
  TargetSelect/23(TargetReplacedCnt) -> Memory30/1
  TargetSelect/1(P0ID) -> [TargetID], P0ID/1
  Memory15/1 -> DeltaDx/1, Product6/1
  [TargetArG] -> Memory28/1
  Memory28/1 -> LostTargetCalc/11(P0ArGK1)
  [TargetRange] -> Memory19/1
  Memory19/1 -> LostTargetCalc/10(P0RangeK1)
  [dyLaneWidthMinHalf] -> Sum11/2, Sum13/2  "dyLaneWidthMinHalf"
  Product6/1 -> Sum13/1
  Sum13/1 -> MinMax4/1
  Gain8/1 -> Product6/2
  Sum11/1 -> Gain8/1
  dyLaneWidthMinHalfStatObj9/1 -> Sum11/1
  [ObjDyc_m] -> TargetSelect/9(Dyc)
  [ObjVyc] -> TargetSelect/10(Vyc)
  [TargetCutIn_b] -> Memory26/1
  [TargetVyc] -> Memory25/1
  [TargetDyc] -> Memory22/1
  [TargetDy] -> Memory21/1
  [TargetDx] -> Memory20/1
  Memory27/1 -> LostTargetCalc/15(tTargetLostK1)
  Memory26/1 -> LostTargetCalc/14(P0CutIn_bK1)
  Memory25/1 -> LostTargetCalc/13(P0VycK1)
  Memory22/1 -> LostTargetCalc/12(P0DycK1)
  Memory21/1 -> LostTargetCalc/9(P0DyK1)
  Memory20/1 -> LostTargetCalc/8(P0DxK1)
  Memory18/1 -> LostTargetCalc/7(P0VxK1)
  [TargetVr] -> Memory18/1
  Memory17/1 -> LostTargetCalc/6(P0IDK1)
  [TargetID] -> Memory17/1
  TargetSelect/21(P0Vyc) -> [TargetVyc]
  TargetSelect/20(P0Dyc) -> [TargetDyc]
  [ObjDy_m] -> LostTargetCalc/3(ObjDy)
  [ObjDx_m] -> LostTargetCalc/2(ObjDx)
  [ObjValid] -> LostTargetCalc/1(ObjValid)
  LostTargetCalc/12(tTargetLost) -> TargetSelect/27(tTargetLost), Memory27/1
  MinMax4/1 -> [dyLaneWidth]
  [ObjSpwLeft] -> TargetSelect/15(spwLeft)
  [ObjSpw] -> TargetSelect/14(spw)
  [ObjwCutIn] -> TargetSelect/13(wCutIn)
  [ObjPlaus] -> TargetSelect/12(plaus)
  TargetSelect/16(P0Dy) -> P0Dy/1, [TargetDy]
  TargetSelect/14(P2Dx) -> P2Dx/1
  TargetSelect/10(P0ArG) -> P0ArG/1, [TargetArG]
  TargetSelect/22(TargetExist) -> TargetExist/1, [TargetExist], Memory24/1
  TargetSelect/19(TargetCutIn_b) -> CutIn_b/1, [TargetCutIn_b]
  [DesireDistanceChar] -> DesireDis/1  "DesireDis"
  TargetSelect/7(P0Vr) -> P0Vr/1, [TargetVr]
  TargetSelect/13(P0Dx) -> P0Dx/1, [TargetDx]
  [ObjDy_m] -> TargetSelect/7(Dy)
  [ObjVy_ms] -> ObjVy_ms/1
  TargetSelect/2(P2ID) -> P2ID/1
  [ObjSpwRight] -> TargetSelect/16(spwRight)
  [Signal_ACC_TgtObjBarDisp] -> Signal_ACC_TgtObjBarDisp/1
  [ObjVx_ms] -> TargetSelect/5(Vr)
  [ObjRange_m] -> TargetSelect/4(Range)
  TargetSelect/15(P3Dx) -> P3Dx/1
  TargetSelect/4(P0Range) -> [TargetRange], P0Range/1
  Memory24/1 -> TargetSelect/33(TargetExistK1)
  [TarLimDx] -> TargetSelect/31(TarLimDx)
  ACCMode1/1 -> TargetSelect/1(ACCmode)
  VxvRef_ms/1 -> TargetSelect/2(vRef)  "OTL_IN_VxvRef_ms_10"
  TargetSelect/3(P3ID) -> P3ID/1
  [ObjValid] -> TargetSelect/3(Valid)
  [ObjClassification] -> TargetSelect/29(Classfication)
  TargetSelect/8(P2Vr) -> P2Vr/1
  TargetSelect/18(P3Dy) -> P3Dy/1
  [ObjArG_ms2] -> TargetSelect/8(ArG)
  [ObjMoveSts] -> TargetSelect/30(MoveSts)
  TargetSelect/11(P2ArG) -> P2ArG/1
  TargetSelect/17(P2Dy) -> P2Dy/1
  [ObjDyc_m] -> ObjDyc_m/1
  TargetSelect/9(P3Vr) -> P3Vr/1
  TargetSelect/12(P3ArG) -> P3ArG/1
  [ObjDx_m] -> TargetSelect/6(Dx)
  Memory14/1 -> Plaus/12(ObjPlausK1)
  Memory13/1 -> Plaus/13(ObjPlausLeftK1)
  Memory6/1 -> Plaus/14(ObjPlausRightK1)
  [ObjLpbRight] -> Plaus/11(ObjLpbRight)
  [ObjLpbLeft] -> Plaus/10(ObjLpbLeft)
  [ObjLpb] -> Plaus/9(ObjLpb)
  [ObjqDycHist] -> Plaus/8(ObjqDycHist)
  [ObjDycHist] -> Plaus/7(ObjDycHist)
  [ObjOnRight] -> Plaus/6(ObjOnRight)
  [ObjOnLeft] -> Plaus/5(ObjOnLeft)
  [ObjVx_ms] -> Plaus/4(ObjVx)
  [ObjDx_m] -> Plaus/3(ObjDx)
  [ObjValid] -> Plaus/2(ObjValid)
  VxvRef_ms_9/1 -> dxMaxFollowPO/1  "OTL_IN_VxvRef_ms_10"
  dxMaxFollowPO/1 -> Plaus/1(dxMaxFollow)
  Plaus/1(ObjPlaus) -> Memory14/1, [ObjPlaus]
  Plaus/2(ObjPlausLeft) -> Memory13/1, [ObjPlausLeft]
  Plaus/3(ObjPlausRight) -> [ObjPlausRight], Memory6/1
  [ObjqDycHist] -> Spw/8(ObjqDycHist)
  [ObjDycHist] -> Spw/7(ObjDycHist)
  [ObjDyc_m] -> Spw/6(ObjDyc)
  Spw/5(ObjOnRight) -> [ObjOnRight]
  Spw/4(ObjOnLeft) -> [ObjOnLeft]
  wCutInVy/4(ObjCutIn_b) -> Terminator20/1
  Spw/3(ObjSpwRight) -> [ObjSpwRight]
  Spw/2(ObjSpwLeft) -> [ObjSpwLeft]
  Spw/1(ObjSpw) -> [ObjSpw]
  [ObjDx_m] -> Spw/5(ObjDx)
  [DycASI] -> Spw/4(DycASI)
  [ObjValid] -> Spw/3(ObjValid)
  [kapCourseErr] -> Spw/2(kapCourseErr)
  alpSumSlideCurveness1/1 -> Spw/1(AlpSumSlideCurveness)
  wCutInVy/1(DycASI) -> [DycASI]
  wCutInVy/3(ObjDycCutInPredict) -> Terminator19/1
  wCutInVy/2(ObjtPrediction4CutIn) -> Terminator18/1
  Memory4/1 -> wCutInVy/9(ObjwCutInVyK1)
  wCutInVy/5(ObjwCutInVy) -> Memory4/1, [ObjwCutIn]
  [ObjDycFilt] -> wCutInVy/8(ObjDycFilt)
  [ObjCnt] -> wCutInVy/7(ObjCnt)
  [ObjDy_m] -> wCutInVy/6(ObjDy)
  [ObjDx_m] -> wCutInVy/5(ObjDx)
  [ObjVyc] -> wCutInVy/4(ObjVyc)
  [ObjWidth_m] -> wCutInVy/3(ObjWidth)
  [ObjDycCutIn] -> wCutInVy/2(ObjDycCutIn)
  [ObjValid] -> wCutInVy/1(ObjValid)
  wCutOutVy/3(ObjwCutOutTurnOff) -> Compare To Constant1/1
  [ObjCnt] -> wCutOutVy/15(ObjCnt)
  [ObjDrive_b] -> wCutOutVy/14(ObjDrive_b)
  [ObjDyc_m] -> wCutOutVy/13(ObjDyc)
  [ObjVy_ms] -> wCutOutVy/12(ObjVy)
  [ObjVx_ms] -> wCutOutVy/11(ObjVx)
  [ObjDy_m] -> wCutOutVy/10(ObjDy)
  dyLaneWidthMinHalfStatObj7/1 -> wCutOutVy/4(tDirIndRight)
  dyLaneWidthMinHalfStatObj5/1 -> wCutOutVy/3(tDirIndLeft)
  VxvRef_ms_8/1 -> wCutOutVy/1(vRef)  "OTL_IN_VxvRef_ms_10"
  kapCurvTraj_4/1 -> wCutOutVy/2(kap)
  wCutOutVy/2(ObjDycCutOutPredict) -> Terminator15/1
  wCutOutVy/1(ObjtPrediction4CutOut) -> Terminator14/1
  Memory2/1 -> wCutOutVy/17(ObjwCutoutVyK1)
  wCutOutVy/4(ObjwCutoutVy) -> Memory2/1, Terminator17/1
  [ObjDycFilt] -> wCutOutVy/16(ObjDycFilt)
  [ObjDx_m] -> wCutOutVy/9(ObjDx)
  [ObjVyc] -> wCutOutVy/8(ObjVyc)
  [ObjWidth_m] -> wCutOutVy/7(ObjWidth)
  [ObjDycCutIn] -> wCutOutVy/6(ObjDycCutIn)
  [ObjValid] -> wCutOutVy/5(ObjValid)
  DycCutIn/2(ObjMove_b) -> [ObjDrive_b]
  Memory1/1 -> DycCutIn/7(dycFiltK1)
  DycCutIn/1(ObjDycCutIn) -> [ObjDycCutIn]
  DycCutIn/3(ObjDycFilt) -> Memory1/1, [ObjDycFilt]
  [ObjqDycHist] -> DycCutIn/6(ObjqDycHist)
  [ObjDycHist] -> DycCutIn/5(ObjDycHist)
  [ObjCnt] -> DycCutIn/4(ObjCnt)
  [ObjMoveSts] -> DycCutIn/3(ObjMoveSts)
  [ObjDyc_m] -> DycCutIn/2(ObjDyc)
  [ObjValid] -> DycCutIn/1(ObjValid)
  [dyLaneWidthLeft] -> Lpb/11(ObjDylaneEdgeLeft)
  [dyEdgeWidthRight] -> Lpb/10(ObjDyEdgeWidthRight)
  [dyEdgeWidthLeft] -> Lpb/12(ObjDyEdgeWidthLeft)
  [dyLaneWidthRight] -> Lpb/9(ObjDylaneEdgeRight)
  Lpb/3(ObjLpbR) -> [ObjLpbRight]
  Lpb/2(ObjLpbL) -> [ObjLpbLeft]
  Lpb/1(ObjLpb) -> [ObjLpb]
  [ObjYawAngle] -> Lpb/8(ObjYawAngle)
  [ObjVyc] -> Lpb/7(ObjVyc)
  [ObjqDycHist] -> Lpb/6(ObjqDycHist)
  [ObjDycHist] -> Lpb/5(ObjDycHist)
  [ObjDyc_m] -> Lpb/4(ObjDyc)
  [ObjValid] -> Lpb/3(ObjValid)
  alpSumSlideCurveness/1 -> Lpb/2(alpSumSlideCurveness)
  VxvRef_ms_1/1 -> Lpb/1(vRef)  "OTL_IN_VxvRef_ms_10"
  VycCalc/2(ObjYawAngle) -> [ObjYawAngle]
  Sum10/1 -> [dyEdgeWidthLeft]  "dyEdgeWidthLeft"
  [dyLaneWidthLeft] -> Sum10/2
  Sum9/1 -> [dyEdgeWidthRight]  "dyEdgeWidthRight"
  Sum8/1 -> Sum10/1, Sum9/2
  [dyLaneWidthRight] -> Sum9/1
  [dyLaneWidthMinHalf] -> Sum8/1
  Product4/1 -> Sum8/2
  [kapCourseErr] -> Product4/2
  Gain4/1 -> Product4/1
  Product3/1 -> Gain4/1
  [ObjDx_m] -> Product3/1, Product3/2
  Dyc/2(kapCourseErr) -> [kapCourseErr]
  Bus Selector1/5 -> VycCalc/5(bP1)  "<bPC1>"
  Bus Selector1/1 -> VycCalc/1(dxC0)  "<dxC0>"
  Bus Selector1/4 -> VycCalc/4(aP1)  "<aPC1>"
  Bus Selector1/2 -> VycCalc/2(aP0)  "<aPC0>"
  Bus Selector1/3 -> VycCalc/3(bP0)  "<bPC0>"
  [EgoLine] -> Bus Selector1/1
  Bus Selector/7 -> DycHistCalc/14(cP1)  "<cPC1>"
  Bus Selector/1 -> DycHistCalc/8(dxC0)  "<dxC0>"
  Bus Selector/6 -> DycHistCalc/13(bP1)  "<bPC1>"
  Bus Selector/2 -> DycHistCalc/9(aP0)  "<aPC0>"
  Bus Selector/5 -> DycHistCalc/12(aP1)  "<aPC1>"
  Bus Selector/3 -> DycHistCalc/10(bP0)  "<bPC0>"
  Bus Selector/4 -> DycHistCalc/11(cP0)  "<cPC0>"
  [EgoLine] -> Bus Selector/1
  VycCalc/1(ObjVyc) -> [ObjVyc]
  [ObjVyG_ms] -> VycCalc/9(ObjVyG)
  [ObjVxG_ms] -> VycCalc/8(ObjVxG)
  [ObjDx_m] -> VycCalc/7(ObjDx)
  [ObjValid] -> VycCalc/6(ObjValid)
  DycHistCalc/2(ObjqDycHist) -> [ObjqDycHist]
  DycHistCalc/1(ObjDycHist) -> [ObjDycHist]
  [ObjValid] -> DycHistCalc/7(ObjValid)
  Bus Creator/1 -> [EgoLine]
  Sum4/1 -> Gain6/1
  Data Type Conversion7/1 -> DesireDistance/1
  Dyc/3(dxC0) -> Bus Creator/1
  Dyc/6(cPC0) -> Bus Creator/4
  Dyc/5(bPC0) -> Bus Creator/3
  Dyc/4(aPC0) -> Bus Creator/2
  ObjValid/1 -> [ObjValid]
  Dyc/8(bPC1) -> Bus Creator/6
  Dyc/7(aPC1) -> Bus Creator/5
  Dyc/9(cPC1) -> Bus Creator/7
  [ObjDx_m] -> Dyc/8(ObjDx)
  [ObjDy_m] -> Dyc/9(ObjDy)
  ObjVyG_ms/1 -> [ObjVyG_ms]
  ObjCnt/1 -> [ObjCnt]
  ObjDy_m/1 -> [ObjDy_m]
  Conf/1 -> Compare To Constant/1
  ObjArG_ms2/1 -> [ObjArG_ms2]
  ObjClassification/1 -> [ObjClassification]
  ObjWidth_m/1 -> [ObjWidth_m]
  ObjVxG_ms/1 -> [ObjVxG_ms]
  ObjMoveSts/1 -> [ObjMoveSts]
  ObjRange_m/1 -> [ObjRange_m]
  AlpWheelAngle/1 -> Abs2/1
  Abs2/1 -> 1-D Lookup Table2/1
  1-D Lookup Table2/1 -> ?  "AlpWheelAngleFactor"
  VxvRef_ms_7/1 -> Dyc/2(vRef)  "OTL_IN_VxvRef_ms_10"
  Compare To Constant/1 -> Dyc/7(LineValid)
  ObjDx_m/1 -> [ObjDx_m]
  kapCurvTraj_1/1 -> Dyc/3(kapTraj)
  AlpSideSlipAngle_1/1 -> Dyc/4(alpSideSlipAngle)
  Dyc/1(kapTrajFilt) -> Memory8/1
  Memory8/1 -> Dyc/1(kapTrajFiltK1)
  [ObjMoveSts] -> Trajectory/7(ObjClass)
  [ObjDy_m] -> Trajectory/6(ObjDy)
  [ObjDx_m] -> Trajectory/5(ObjDx)
  [ObjCnt] -> Trajectory/8(ObjCntAlive)
  [ObjValid] -> Trajectory/4(ObjValid)
  VxvRef_ms_6/1 -> Trajectory/2(VxvRef)  "OTL_IN_VxvRef_ms_10"
  AlpSideSlipAngle/1 -> Trajectory/3(AlpSideSlipAngle)
  kapCurvTraj_2/1 -> Trajectory/1(Kap)
  kapCurvTraj_3/1 -> VxVy/2(Kap)
  [ObjVxG_ms] -> VxVy/3(VxG)
  [ObjVyG_ms] -> VxVy/4(VyG)
  VxVy/2(Vy) -> [ObjVy_ms]
  VxVy/1(Vx) -> [ObjVx_ms]
  VxvRef_ms_5/1 -> VxVy/1(VxvRef)  "OTL_IN_VxvRef_ms_10"
  Sum3/1 -> Gain2/1
  MinMax2/1 -> Sum4/1, Sum3/1
  dyLaneWidthMinHalfStatObj2/1 -> Sum1/1, MinMax2/2
  Sum2/1 -> MinMax2/1
  Product2/1 -> Sum2/1
  [ObjDx_m] -> Product2/1
  Gain5/1 -> Product2/2
  Sum1/1 -> Gain5/1
  MinMax1/1 -> Sum4/2  "dyLaneWidthSteerAdaptRight"
  MinMax/1 -> Sum3/2  "dyLaneWidthSteerAdaptLeft"
  dyLaneWidthSteerAdapt/2(dyLaneAdaptRight) -> MinMax1/2
  dyLaneWidthSteerAdapt/1(dyLaneAdaptLeft) -> MinMax/2
  t_dyLaneWidthSteerAdapt/1 -> MinMax/1, MinMax1/1
  Abs1/1 -> t_dyLaneWidthSteerAdapt/1
  Abs/1 -> dyLaneWidthSteerAdapt/2(dyAdapt)  "dyAdapt"
  Product1/1 -> Abs/1
  Gain3/1 -> Product1/2
  Product/1 -> Product1/1
  kapCurvTraj/1 -> dyLaneWidthSteerAdapt/1(kap), Product/1, Abs1/1
  dyLaneWidthMinHalfStatObj1/1 -> Gain3/1, Product/2
  Gain/1 -> Sum1/2, Sum2/2, [dyLaneWidthMinHalf]  "dyLaneWidthMinHalf"
  dyLaneWidthMin/1 -> Gain/1
  VxvRef_ms_3/1 -> dyLaneWidthMin/1  "OTL_IN_VxvRef_ms_10"
  TimeGap/1 -> Data Type Conversion7/1, ACC_DisplayBar/1(TimeGap)
  ACCMode/1 -> ACC_DisplayBar/3(ACCmode)
  [TargetExist] -> ACC_DisplayBar/6(TargetExist)
  [TargetRange] -> ACC_DisplayBar/4(TargetRange)
  ACC_DisplayBar/1(DisplayBar) -> Memory10/1, [Signal_ACC_TgtObjBarDisp]
  Constant3/1 -> ACC_DisplayBar/5(Scale)
  Memory10/1 -> ACC_DisplayBar/7(DisplayBarK1)
  DesireDistance/1 -> [DesireDistanceChar]
  Dyc/10(ObjDyc) -> [ObjDyc_m]

== system Noa_Nofusion_backup/Subsystem2/ACCOSM/ObjMatrixTransit ==
  EQ4_OBJ : Inport
  Bus Creator : BusCreator  Inputs=14
  Bus Selector4 : BusSelector  OutputSignals=EQ4_OBJ_HDR.OBJ_Sync_ID,EQ4_OBJ_HDR.OBJ_VRU_Count,EQ4_OBJ_HDR.OBJ_VD_Count,EQ4_OBJ_HDR.OBJ_General_OBJ_Count,EQ4_OBJ_HDR.OBJ_Animal_Count,EQ4_OBJ_ELEM
  Data Type Conversion : DataTypeConversion
  IFV2FrontBumper : Constant  Value=1.7  OutDataTypeStr=single
  IFV2RearAxis : Constant  Value=2.1  OutDataTypeStr=single
  Subsystem : Subsystem
  Sum : Sum  Inputs=++++
  Sum1 : Sum  Inputs=|-+
  Sum5 : Sum  Inputs=++|
  Terminator1 : Terminator
  VisObjSts : Outport
  wires:
  Subsystem/6(ObjLatVel) -> Bus Creator/7  "ObjLatVel"
  Subsystem/4(ObjClassification) -> Bus Creator/5  "ObjClassification"
  Subsystem/2(ObjValid) -> Bus Creator/3  "ObjValid"
  Subsystem/7(ObjLongAccel) -> Bus Creator/8  "ObjLongAccel"
  Subsystem/5(ObjLatPos) -> Bus Creator/6  "ObjLatPos"
  Subsystem/3(ObjBrakeLightIndic) -> Bus Creator/4  "ObjBrakeLightIndic"
  Subsystem/9(ObjWidth) -> Bus Creator/10  "ObjWidth"
  Subsystem/12(ObjLongPos) -> Sum1/2, Sum5/1
  Subsystem/8(ObjLongVel) -> Bus Creator/9  "ObjLongVel"
  Subsystem/10(ObjCnt) -> Bus Creator/11  "ObjCnt"
  Sum1/1 -> Bus Creator/13  "ObjRange_m"
  Subsystem/11(ObjMoveSts) -> Bus Creator/12  "ObjMoveSts"
  Sum5/1 -> Bus Creator/14  "ObjDx_m"
  IFV2RearAxis/1 -> Sum5/2
  Data Type Conversion/1 -> Bus Creator/1  "Cnt"
  IFV2FrontBumper/1 -> Sum1/1
  Bus Creator/1 -> VisObjSts/1  "ObjSts"
  Subsystem/1(ObjID) -> Bus Creator/2  "ObjID"
  Bus Selector4/6 -> Subsystem/2(<EQ4_OBJ_ELEM>)  "<EQ4_OBJ_ELEM>"
  Sum/1 -> Subsystem/1(Count)
  Bus Selector4/4 -> Sum/3  "<OBJ_General_OBJ_Count>"
  Bus Selector4/3 -> Sum/2  "<OBJ_VD_Count>"
  Bus Selector4/2 -> Sum/1  "<OBJ_VRU_Count>"
  Bus Selector4/1 -> Data Type Conversion/1  "<OBJ_Sync_ID>"
  Bus Selector4/5 -> Sum/4  "<OBJ_Animal_Count>"
  EQ4_OBJ/1 -> Bus Selector4/1
  Subsystem/13(P) -> Terminator1/1

== system Noa_Nofusion_backup/Subsystem2/ACCOSM/rollingcounter 1 ==
  Constant7 : Constant  OutDataTypeStr=Inherit: Inherit via back propagation
  Constant8 : Constant  Value=7  OutDataTypeStr=Inherit: Inherit via back propagation
  Constant9 : Constant  Value=0  OutDataTypeStr=Inherit: Inherit via back propagation
  Relational Operator : RelationalOperator  Operator=>  OutDataTypeStr=boolean  RndMeth=Nearest
  Sum : Sum  Inputs=|++
  Switch : Switch  Criteria=u2 ~= 0  Threshold=1
  Unit Delay : UnitDelay  SampleTime=-1  HasFrameUpgradeWarning=on
  cnt : Outport
  wires:
  Constant9/1 -> Switch/1
  Sum/1 -> Switch/3, Relational Operator/1
  Constant8/1 -> Relational Operator/2
  Unit Delay/1 -> Sum/2
  Constant7/1 -> Sum/1
  Relational Operator/1 -> Switch/2
  Switch/1 -> cnt/1, Unit Delay/1
